simulink model "actividad1"  (R2021a)
settings: Solver=VariableStepAuto  StartTime=0.0  StopTime=2  FixedStep=1e-5  RelTol=1e-3
libraries: pid_lib x1
settings Model: Creator=Agus  LastModifiedBy=valen

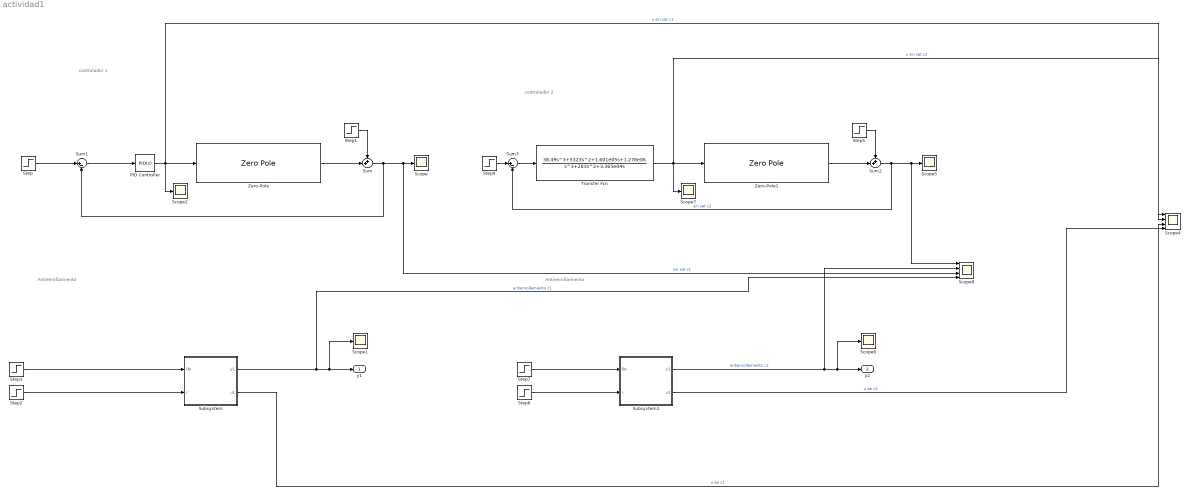
== system actividad1 ==
  note: controlador 2
  note: controlador 1
  note: Antienrollamiento
  note: Antienrollamiento
  PID Controller : pid_lib/PID Controller  Controller=PID  Form=Parallel  TimeDomain=Continuous-time  UseExternalTs=off  SampleTime=-1  IntegratorMethod=Forward Euler  FilterMethod=Forward Euler  ControllerParametersSource=internal  P=2.1595  I=8.175  D=0.0733  UseFilter=on  N=1364.25  TunerSelectOption=Transfer Function Based (PID Tuner App)  InitialConditionSource=internal  InitialConditionForIntegrator=0  InitialConditionForFilter=0  DifferentiatorICPrevScaledInput=0  ExternalReset=none  TrackingMode=off  Kt=1  LimitOutput=off  SatLimitsSource=internal  UpperSaturationLimit=inf  LowerSaturationLimit=-inf  LinearizeAsGain=on  AntiWindupMode=none  Kb=1  POutMin=[]  POutMax=[]  IOutMin=[]  IOutMax=[]  DOutMin=[]  DOutMax=[]  NOutMin=[]  NOutMax=[]  SumOutMin=[]  SumOutMax=[]  SaturationOutMin=[]  SaturationOutMax=[]  PParamMin=[]  PParamMax=[]  IParamMin=[]  IParamMax=[]  DParamMin=[]  DParamMax=[]  NParamMin=[]  NParamMax=[]  KbParamMin=[]  KbParamMax=[]  KtParamMin=[]  KtParamMax=[]  KbOutMin=[]  KbOutMax=[]  KtOutMin=[]  KtOutMax=[]  IntegratorOutMin=[]  IntegratorOutMax=[]  FilterOutMin=[]  FilterOutMax=[]  SumI1OutMin=[]  SumI1OutMax=[]  SumI2OutMin=[]  SumI2OutMax=[]  SumI3OutMin=[]  SumI3OutMax=[]  SumI4OutMin=[]  SumI4OutMax=[]  SumDOutMin=[]  SumDOutMax=[]  DifferentiatorOutMin=[]  DifferentiatorOutMax=[]  FilterDiffOutCoefMin=[]  FilterDiffOutCoefMax=[]  ReciprocalOutMin=[]  ReciprocalOutMax=[]  SumDenOutMin=[]  SumDenOutMax=[]  SumNumOutMin=[]  SumNumOutMax=[]  DivideOutMin=[]  DivideOutMax=[]  UdiffTsProdOutMin=[]  UdiffTsProdOutMax=[]  NTsProdOutMin=[]  NTsProdOutMax=[]  UintegralTsProdOutMin=[]  UintegralTsProdOutMax=[]  UngainTsProdOutMin=[]  UngainTsProdOutMax=[]  IntegratorContinuousStateAttributes=''  IntegratorStateMustResolveToSignalObject=off  IntegratorRTWStateStorageClass=Auto  FilterContinuousStateAttributes=''  FilterStateMustResolveToSignalObject=off  FilterRTWStateStorageClass=Auto  ParallelPVariant=InternalParameters  IdealPVariant=Disabled  IVariant=InternalParameters  DVariant=InternalParameters  IntegratorVariant=Continuous  SatVariant=Disabled  AWVariant=Passthrough  PCopyVariant=Disabled  TRVariant=Disabled  FdbkBlocksVariant=Forward  IdealPFdbkVariant=Disabled  SatFdbkVariant=Disabled  DerivativeFilterVariant=ContFilter  NVariant=InternalParameters  NCopyVariant=Disabled  FilterICVariant=InternalICsFilter  IntegratorICVariant=InternalICs  ExternalResetVariant=Disabled  TRSumVariant=Passthrough  SumFdbkVariant=Disabled  SumVariant=Sum_PID  TsampFilterVariant=InternalTs  TsampNgainVariant=Passthrough  TsampIntegralVariant=Passthrough  ExternalSaturationOutDataTypeStr=Inherit: Same as second input
  Scope{,1..2,5..7} (6 alike) : Scope
  Scope4 : Scope  NumInputPorts=4
  Scope9 : Scope  NumInputPorts=4
  Step{,2,4,6} (4 alike) : Step  Time=0  After=-1  SampleTime=0
  Step{1,3,5,7} (4 alike) : Step  SampleTime=0
  Subsystem : Subsystem  mask{Ki=8.175, Kp=2.1595, Kd=0.0733, tau=7.33e-4, sat=10}
  Subsystem1 : Subsystem  mask{Ki=8.175, Kp=2.1595, Kd=0.0733, tau=7.33e-4, sat=10}
  Sum : Sum  Inputs=++|
  Sum1 : Sum  Inputs=|+-
  Sum2 : Sum  Inputs=++|
  Sum3 : Sum  Inputs=|+-
  Transfer Fcn : TransferFcn  Numerator=[38.49 5323 1.601e05 1.278e06]  Denominator=[1 283 3.365e04 0]
  Zero-Pole : ZeroPole  Zeros=[]  Poles=[-100 -25 +25]  Gain=[57500]
  Zero-Pole1 : ZeroPole  Zeros=[]  Poles=[-100 -25 +25]  Gain=[57500]
  y1 : Outport
  y2 : Outport  Port=2
  wires:
  PID Controller/1 -> Scope2/1, Scope4/2, Zero-Pole/1  "u sin sat c1"
  Zero-Pole/1 -> Sum/2
  Step1/1 -> Sum/1
  Sum1/1 -> PID Controller/1
  Step/1 -> Sum1/1
  Sum/1 -> Scope9/3, Scope/1, Sum1/2  "sin sat c1"
  Step3/1 -> Subsystem/1(Do)
  Step2/1 -> Subsystem/2(r)
  Subsystem/1(y1) -> Scope9/4, Scope1/1, y1/1  "antienrollamiento c1"
  Subsystem/2(u1) -> Scope4/3  "u ae c1"
  Transfer Fcn/1 -> Scope7/1, Scope4/1, Zero-Pole1/1  "u sin sat c2"
  Sum2/1 -> Scope9/1, Scope5/1, Sum3/2  "sin sat c2"
  Step7/1 -> Subsystem1/1(Do)
  Subsystem1/1(y1) -> Scope9/2, Scope6/1, y2/1  "antienrollamiento c2"
  Step5/1 -> Sum2/1
  Zero-Pole1/1 -> Sum2/2
  Step6/1 -> Subsystem1/2(r)
  Subsystem1/2(u1) -> Scope4/4  "u ae c2"
  Step4/1 -> Sum3/1
  Sum3/1 -> Transfer Fcn/1

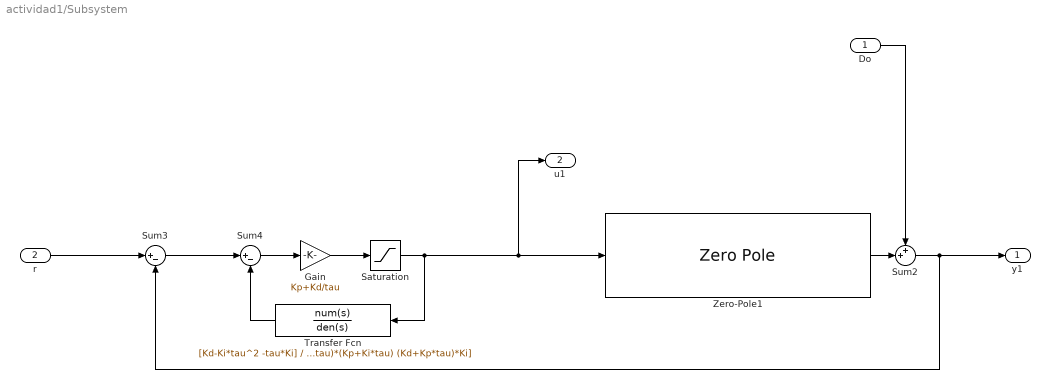
== system actividad1/Subsystem ==
  Do : Inport
  r : Inport  Port=2
  Gain : Gain  Gain=Kp+Kd/tau
  Saturation : Saturate  UpperLimit=sat  LowerLimit=-sat
  Sum2 : Sum  Inputs=++|
  Sum3 : Sum  Inputs=|+-
  Sum4 : Sum  Inputs=|+-
  Transfer Fcn : TransferFcn  Numerator=[Kd-Ki*tau^2 -tau*Ki]  Denominator=[(Kd+Kp*tau)^2 (Kd+Kp*tau)*(Kp+Ki*tau) (Kd+Kp*tau)*Ki]
  Zero-Pole1 : ZeroPole  Zeros=[]  Poles=[-100 -25 +25]  Gain=[57500]
  y1 : Outport
  u1 : Outport  Port=2
  wires:
  Sum3/1 -> Sum4/1
  Zero-Pole1/1 -> Sum2/2
  Gain/1 -> Saturation/1
  Saturation/1 -> u1/1, Zero-Pole1/1, Transfer Fcn/1
  Sum2/1 -> y1/1, Sum3/2
  r/1 -> Sum3/1
  Transfer Fcn/1 -> Sum4/2
  Do/1 -> Sum2/1
  Sum4/1 -> Gain/1

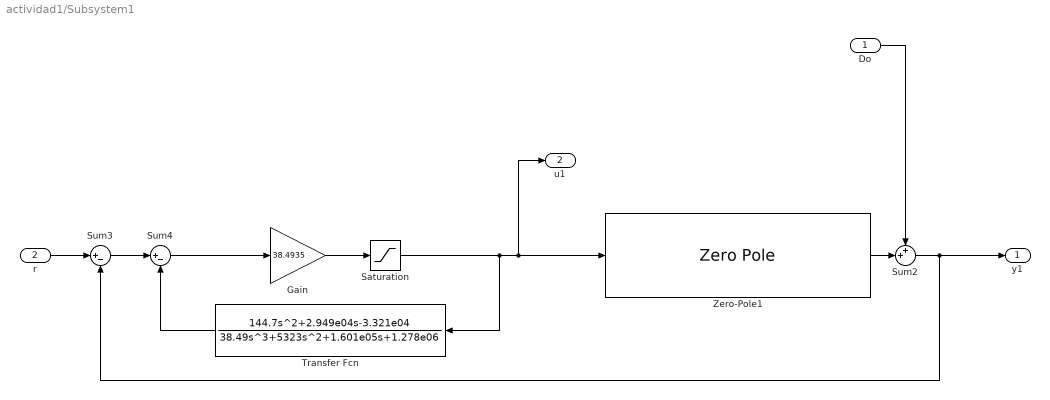
== system actividad1/Subsystem1 ==
  Do : Inport
  r : Inport  Port=2
  Gain : Gain  Gain=38.4935
  Saturation : Saturate  UpperLimit=sat  LowerLimit=-sat
  Sum2 : Sum  Inputs=++|
  Sum3 : Sum  Inputs=|+-
  Sum4 : Sum  Inputs=|+-
  Transfer Fcn : TransferFcn  Numerator=[144.7 2.949e04 -3.321e04]  Denominator=[38.49 5323 1.601e05 1.278e06]
  Zero-Pole1 : ZeroPole  Zeros=[]  Poles=[-100 -25 +25]  Gain=[57500]
  y1 : Outport
  u1 : Outport  Port=2
  wires:
  Sum3/1 -> Sum4/1
  Zero-Pole1/1 -> Sum2/2
  Gain/1 -> Saturation/1
  Saturation/1 -> u1/1, Zero-Pole1/1, Transfer Fcn/1
  Sum2/1 -> y1/1, Sum3/2
  r/1 -> Sum3/1
  Transfer Fcn/1 -> Sum4/2
  Do/1 -> Sum2/1
  Sum4/1 -> Gain/1
